simulink model "KSimulator_robotExM1_NPC"  (Simulink 9.0)
settings: Solver=FixedStepDiscrete  StartTime=0.0  StopTime=10  FixedStep=0.01  RelTol=1e-3  EnableMultiTasking=on
undefined symbols (not defined in the file or in its folder): SimpleRobotPlot
settings Model: SuppressorTable=22 serialization::archive 11 0 6 0 0 0 11 0  Creator=E. Dean  LastModifiedBy=nirnai
settings DataIOCC: LimitDataPoints=on  SignalLoggingSaveFormat=ModelDataLogs
settings OptimizationCC: ExpressionDepthLimit=2147483647
settings DebuggingCC: SolverPrmCheckMsg=warning  FcnCallInpInsideContextMsg=warning  StateNameClashWarn=warning
settings GRTTargetCC: GeneratePreprocessorConditionals=Disable all  CombineOutputUpdateFcns=off  GRTInterface=on

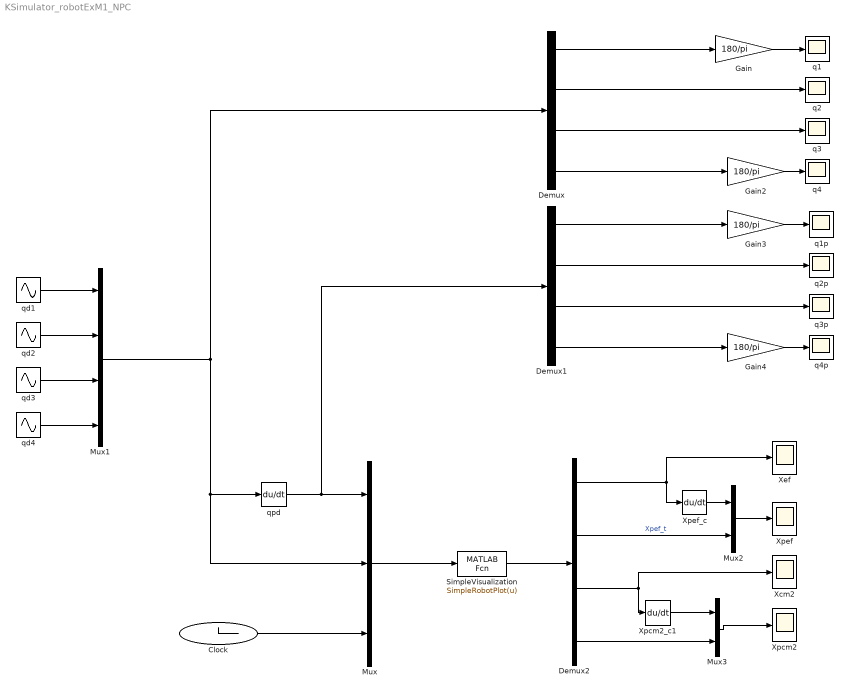
== system KSimulator_robotExM1_NPC ==
  Clock : Clock
  Demux : Demux
  Demux1 : Demux
  Demux2 : Demux
  Gain{,2..4} (4 alike) : Gain  Gain=180/pi
  Mux : Mux  Inputs=3
  Mux1 : Mux
  Mux2 : Mux  Inputs=2
  Mux3 : Mux  Inputs=2
  SimpleVisualization : MATLABFcn  MATLABFcn=SimpleRobotPlot(u)  OutputDimensions=12
  Xcm2 : Scope
  Xef : Scope
  Xpcm2 : Scope
  Xpcm2_c1 : Derivative
  Xpef : Scope
  Xpef_c : Derivative
  q{1..4} (4 alike) : Scope
  q1p : Scope
  q2p : Scope
  q3p : Scope
  q4p : Scope
  qd1 : Sin  Amplitude=pi/2  SampleTime=0
  qd2 : Sin  Amplitude=0.04  Bias=0.06  SampleTime=0
  qd3 : Sin  Amplitude=0.04  Bias=0.06  SampleTime=0
  qd4 : Sin  Amplitude=pi/2  SampleTime=0
  qpd : Derivative
  wires:
  Demux/1 -> Gain/1
  Demux/2 -> q2/1
  Mux/1 -> SimpleVisualization/1
  Demux/3 -> q3/1
  qd1/1 -> Mux1/1
  qd2/1 -> Mux1/2
  qd3/1 -> Mux1/3
  Mux1/1 -> Demux/1, qpd/1, Mux/2
  Demux1/2 -> q2p/1
  Demux1/3 -> q3p/1
  Demux1/1 -> Gain3/1
  qpd/1 -> Demux1/1, Mux/1
  SimpleVisualization/1 -> Demux2/1
  Demux2/1 -> Xef/1, Xpef_c/1
  Mux2/1 -> Xpef/1
  Xpef_c/1 -> Mux2/1
  Demux2/2 -> Mux2/2  "Xpef_t"
  Demux2/3 -> Xcm2/1, Xpcm2_c1/1
  Mux3/1 -> Xpcm2/1
  Xpcm2_c1/1 -> Mux3/1
  Demux2/4 -> Mux3/2
  qd4/1 -> Mux1/4
  Demux/4 -> Gain2/1
  Demux1/4 -> Gain4/1
  Gain2/1 -> q4/1
  Gain/1 -> q1/1
  Gain4/1 -> q4p/1
  Gain3/1 -> q1p/1
  Clock/1 -> Mux/3
